simulink model "CubeX"  (R2016b)
settings: Solver=FixedStepAuto  StartTime=0.0  StopTime=10.0  RelTol=1e-3
values from neighbouring files (symbols this model uses):
  A = [0 0 0 0 0 0 0 0 0 0 283.190307038 0 ... (36 elements, 6x6)]    [K_lqr_3D.mat]
  C = [1 0 0 0 0 0 0 1 0 0 0 0 ... (36 elements, 6x6)]    [K_lqr_3D.mat]
  controller =     [K_lqr_3D.mat]
  deg_ = 0.0174532925199    [K_lqr_3D.mat]
  g = 9.81    [K_lqr_3D.mat]
  imu =     [K_lqr_3D.mat]
  K_lqr = [204.402503892 25.7626324054]    [K_lqr_3D.mat]
undefined symbols (not defined in the file or in its folder): CPHA_1Edge, CPOL_Low, Duplex, FirstBit_MSB, Full, Link, LQFP100, ST, STM32F407VG, STM32F4DISCOVERY
libraries: simulink x22, stm32f4_spi_lib x4, stm32f4_io_lib x2, stm32f4_adc_lib x1, cube_lib x1, stm32f4_device_config_lib x1, BC_USB x1
(part 2 of 3)

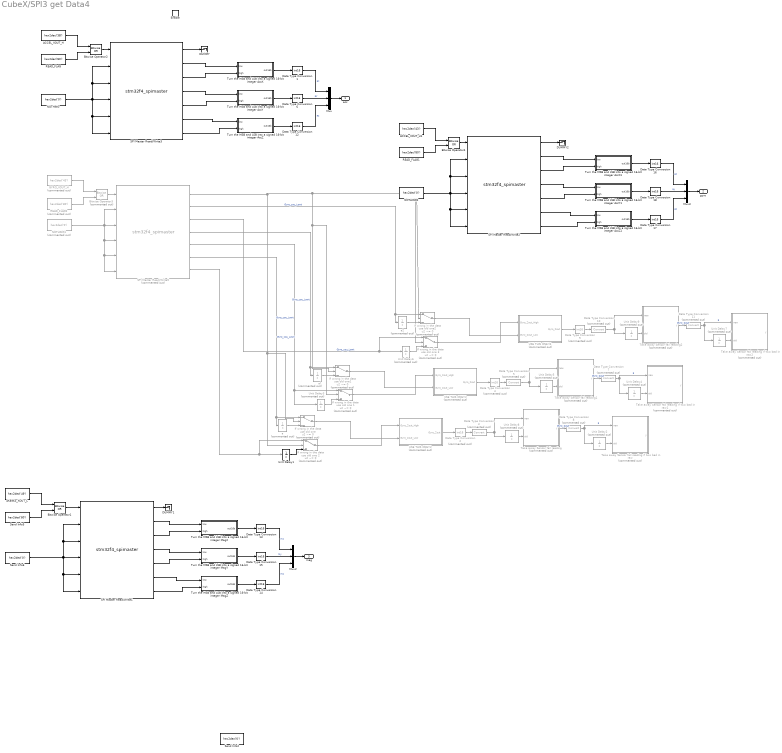
== system CubeX/SPI3 get Data4 ==
  Enable : EnablePort
  " a" : UnitDelay  Commented=on  SampleTime=-1
  " a1" : UnitDelay  Commented=on  SampleTime=-1
  " a2" : UnitDelay  Commented=on  SampleTime=-1
  ACCEL_XOUT_H : Constant  Value=hex2dec('3B')  OutDataTypeStr=uint8
  ACCEL_XOUT_H1 : Constant  Value=hex2dec('43')  OutDataTypeStr=uint8
  AK8963_XOUT_L : Constant  Value=hex2dec('49')  OutDataTypeStr=uint8
  Bitwise Operator1 : simulink/Logic and Bit Operations/Bitwise Operator  logicop=OR  UseBitMask=off  NumInputPorts=2  BitMask=bin2dec('11011001')  BitMaskRealWorld=Stored Integer
  Bitwise Operator2 : simulink/Logic and Bit Operations/Bitwise Operator  logicop=OR  UseBitMask=off  NumInputPorts=2  BitMask=bin2dec('11011001')  BitMaskRealWorld=Stored Integer
  Bitwise Operator3 : simulink/Logic and Bit Operations/Bitwise Operator  Commented=on  logicop=OR  UseBitMask=off  NumInputPorts=2  BitMask=bin2dec('11011001')  BitMaskRealWorld=Stored Integer
  Bitwise Operator4 : simulink/Logic and Bit Operations/Bitwise Operator  logicop=OR  UseBitMask=off  NumInputPorts=2  BitMask=bin2dec('11011001')  BitMaskRealWorld=Stored Integer
  DUMMY : Terminator
  DUMMY1 : Terminator
  DUMMY2 : Terminator
  Data Type Conversion{1,6,12..18} (9 alike) : DataTypeConversion  OutDataTypeStr=int16
  Data Type Conversion{3,5,7..8,10..11} (6 alike) : DataTypeConversion  Commented=on
  Data Type Conversion2 : DataTypeConversion  Commented=on  OutDataTypeStr=int16
  Data Type Conversion4 : DataTypeConversion  Commented=on  OutDataTypeStr=int16
  Data Type Conversion9 : DataTypeConversion  Commented=on  OutDataTypeStr=int16
  GYRO_XOUT_H : Constant  Commented=on  Value=hex2dec('43')  OutDataTypeStr=uint8
  If wrong in the data use old one : Switch  Commented=on  Criteria=u2 ~= 0
  If wrong in the data use old one 1 : Switch  Commented=on  Criteria=u2 ~= 0
  If wrong in the data use old one 2 : Switch  Commented=on  Criteria=u2 ~= 0
  If wrong in the data use old one 3 : Switch  Commented=on  Criteria=u2 ~= 0
  If wrong in the data use old one1 : Switch  Commented=on  Criteria=u2 ~= 0
  If wrong in the data use old one2 : Switch  Commented=on  Criteria=u2 ~= 0
  Mux : Mux  Inputs=3
  Mux2 : Mux  Inputs=3
  Mux3 : Mux  Inputs=3
  NOTHING : Constant  Value=hex2dec('0')  OutDataTypeStr=uint8
  NOTHING1 : Constant  Commented=on  Value=hex2dec('0')  OutDataTypeStr=uint8
  NOTHING2 : Constant  Value=hex2dec('0')  OutDataTypeStr=uint8
  READ_FLAG : Constant  Value=hex2dec('80')  OutDataTypeStr=uint8
  READ_FLAG1 : Constant  Value=hex2dec('80')  OutDataTypeStr=uint8
  READ_FLAG2 : Constant  Commented=on  Value=hex2dec('80')  OutDataTypeStr=uint8
  SPI Master Read/Write1 : S-Function  FunctionName=stm32f4_spimaster  Parameters=mode,configuration,module,datacount,inputtypearray,outputtypearray,confstr,sampletime,sampletimestr,blockid  SFunctionDeploymentMode=off  EnableBusSupport=off  mask(stm32f4_spimaster){configuration=Transaction, module=3, mode=Read/ Write, lastmodule=1, direction=Full-Duplex, dataformat=8bit/ FirstBit_MSB, prescaler=4, cpolcpha=CPOL_Low/ CPHA_1Edge, datacount=6, nssmode=Custom, nsspin=Not used, softnssport=E, softnsspin=0, sckpin=A5, misopin=A6, mosipin=A7, inputtypearray=[6 3 3 3 3 3 3], outputtypearray=[7 7 3 3 3 3 3 3], confstr=["SPI_Direction_2Lines_FullDuplex","8b","MSB","Low","1Edge","4","Soft","0","x","x","0","x","x","1","A","5","1","A","6","1","A","7","1","0","0","0","0","0","0","0","0","PP","0","UP"], sampletime=0.002, sampletimestr=0.002, blockid=SPI3getData4SPIMasterReadWrite1}
      mask prompts: module "SPI Module:"; lastmodule "Last module:"; dataformat "Data format:"; prescaler "Buad rate prescaler: Pclk/"; cpolcpha "Clock polarity (CPOL)/ Clock phase (CPHA):"; datacount "Data Read/Write count:"; nssmode "Slave/chip select (nSS, nCS) mode"; nsspin "Slave/chip select (nSS, nCS) pin"; softnssport "Slave/chip select port (nSS, nCS)"; softnsspin "Slave/chip select pin (nSS, nCS)"; sckpin "SCLK pin:"; misopin "MISO pin:"; mosipin "MOSI pin:"; inputtypearray "Input type array"; outputtypearray "Output type array"; confstr "Configuration string"; sampletime "Sample time (sec)"; sampletimestr "Compiled sample time (sec) in string"
      mask help:
      | Status:
      |  0 - Success.
      |  Otherwise - Fail.
      mask init:
      | stm32f4_spimaster_callback('init');
      mask Help: web(fullfile(waijungdocroot,'stm32f4_spimaster_readwrite.htm'), '-browser')
      mask TypeOptions configuration: Setup | Transaction
      mask Callback configuration: stm32f4_spimaster_callback('configuration');
      mask TypeOptions module: 1 | 2 | 3
      mask Callback module: stm32f4_spimaster_callback('module');
      mask TypeOptions mode: Read/ Write | Read | Write
      mask Callback mode: stm32f4_spimaster_callback('mode');
      mask TypeOptions direction: Full-Duplex | Half-Duplex_Tx | Half-Duplex_Rx
      mask Callback direction: stm32f4_spimaster_callback('direction');
      mask TypeOptions dataformat: 8bit/ FirstBit_MSB | 8bit/ FirstBit_LSB | 16bit/ FirstBit_MSB | 16bit/ FirstBit_LSB
      mask TypeOptions prescaler: 2 | 4 | 8 | 16 | 32 | 64 | 128 | 256
      mask TypeOptions cpolcpha: CPOL_Low/ CPHA_1Edge | CPOL_Low/ CPHA_2Edge | CPOL_High/ CPHA_1Edge | CPOL_High/ CPHA_2Edge
      mask Callback datacount: stm32f4_spimaster_callback('datacount');
      mask TypeOptions nssmode: Hardware | Software | Custom
      mask Callback nssmode: stm32f4_spimaster_callback('nssmode');
      mask TypeOptions nsspin: Not used | A4 | A15
      mask TypeOptions softnssport: A | B | C | D | E | F | G | H | I
      mask TypeOptions softnsspin: 0 | 1 | 2 | 3 | 4 | 5 | 6 | 7 | 8 | 9 | 10 | 11 | 12 | 13 | 14 | 15
      mask TypeOptions sckpin: Not used | A5 | B3
      mask TypeOptions misopin: Not used | A6 | B4
      mask TypeOptions mosipin: Not used | A7 | B5
      mask Callback confstr: stm32f4_spimaster_callback('confstr');
      mask Callback sampletime: stm32f4_spimaster_callback('sampletime');
      mask Callback sampletimestr: stm32f4_spimaster_callback('sampletimestr');
      mask Callback blockid: stm32f4_spimaster_callback('blockid');
      mask Display: text(0.5, 0.5, 'Module: SPI3 (Master)\nRead/ Write\nTs (sec): 0.002','ver','middle','hor','center');port_label('input', 1,'Wr0 (uint8)');port_label('input', 2,'Wr1 (uint8)');port_label('input', 3,'Wr2 (uint8)');port_label('input', 4,'Wr3 (uint8)');port_label('input', 5,'Wr4 (uint8)');port_label('input', 6,'Wr5 (uint8)');port_label('output', 1,'Status');port_label('output', 2,'Rd0 (uint8)');port_label('output', 3,'Rd1 (uint8)');port_label('output', 4,'Rd2 (uint8)');port_label('output', 5,'Rd3 (uint8)');port_label('output', 6,'Rd4 (uint8)');port_label('output', 7,'Rd5 (uint8)');
  SPI Master Read/Write2 : S-Function  FunctionName=stm32f4_spimaster  Parameters=mode,configuration,module,datacount,inputtypearray,outputtypearray,confstr,sampletime,sampletimestr,blockid  SFunctionDeploymentMode=off  EnableBusSupport=off  mask(stm32f4_spimaster){configuration=Transaction, module=3, mode=Read/ Write, lastmodule=1, direction=Full-Duplex, dataformat=8bit/ FirstBit_MSB, prescaler=4, cpolcpha=CPOL_Low/ CPHA_1Edge, datacount=6, nssmode=Custom, nsspin=Not used, softnssport=E, softnsspin=0, sckpin=A5, misopin=A6, mosipin=A7, inputtypearray=[6 3 3 3 3 3 3], outputtypearray=[7 7 3 3 3 3 3 3], confstr=["SPI_Direction_2Lines_FullDuplex","8b","MSB","Low","1Edge","4","Soft","0","x","x","0","x","x","1","A","5","1","A","6","1","A","7","1","0","0","0","0","0","0","0","0","PP","0","UP"], sampletime=-1, sampletimestr=Inf, blockid=SPI3getData4SPIMasterReadWrite2}
      mask prompts: module "SPI Module:"; lastmodule "Last module:"; dataformat "Data format:"; prescaler "Buad rate prescaler: Pclk/"; cpolcpha "Clock polarity (CPOL)/ Clock phase (CPHA):"; datacount "Data Read/Write count:"; nssmode "Slave/chip select (nSS, nCS) mode"; nsspin "Slave/chip select (nSS, nCS) pin"; softnssport "Slave/chip select port (nSS, nCS)"; softnsspin "Slave/chip select pin (nSS, nCS)"; sckpin "SCLK pin:"; misopin "MISO pin:"; mosipin "MOSI pin:"; inputtypearray "Input type array"; outputtypearray "Output type array"; confstr "Configuration string"; sampletime "Sample time (sec)"; sampletimestr "Compiled sample time (sec) in string"
      mask help:
      | Status:
      |  0 - Success.
      |  Otherwise - Fail.
      mask init:
      | stm32f4_spimaster_callback('init');
      mask Help: web(fullfile(waijungdocroot,'stm32f4_spimaster_readwrite.htm'), '-browser')
      mask TypeOptions configuration: Setup | Transaction
      mask Callback configuration: stm32f4_spimaster_callback('configuration');
      mask TypeOptions module: 1 | 2 | 3
      mask Callback module: stm32f4_spimaster_callback('module');
      mask TypeOptions mode: Read/ Write | Read | Write
      mask Callback mode: stm32f4_spimaster_callback('mode');
      mask TypeOptions direction: Full-Duplex | Half-Duplex_Tx | Half-Duplex_Rx
      mask Callback direction: stm32f4_spimaster_callback('direction');
      mask TypeOptions dataformat: 8bit/ FirstBit_MSB | 8bit/ FirstBit_LSB | 16bit/ FirstBit_MSB | 16bit/ FirstBit_LSB
      mask TypeOptions prescaler: 2 | 4 | 8 | 16 | 32 | 64 | 128 | 256
      mask TypeOptions cpolcpha: CPOL_Low/ CPHA_1Edge | CPOL_Low/ CPHA_2Edge | CPOL_High/ CPHA_1Edge | CPOL_High/ CPHA_2Edge
      mask Callback datacount: stm32f4_spimaster_callback('datacount');
      mask TypeOptions nssmode: Hardware | Software | Custom
      mask Callback nssmode: stm32f4_spimaster_callback('nssmode');
      mask TypeOptions nsspin: Not used | A4 | A15
      mask TypeOptions softnssport: A | B | C | D | E | F | G | H | I
      mask TypeOptions softnsspin: 0 | 1 | 2 | 3 | 4 | 5 | 6 | 7 | 8 | 9 | 10 | 11 | 12 | 13 | 14 | 15
      mask TypeOptions sckpin: Not used | A5 | B3
      mask TypeOptions misopin: Not used | A6 | B4
      mask TypeOptions mosipin: Not used | A7 | B5
      mask Callback confstr: stm32f4_spimaster_callback('confstr');
      mask Callback sampletime: stm32f4_spimaster_callback('sampletime');
      mask Callback sampletimestr: stm32f4_spimaster_callback('sampletimestr');
      mask Callback blockid: stm32f4_spimaster_callback('blockid');
      mask Display: text(0.5, 0.5, 'Module: SPI3 (Master)\nRead/ Write\nTs (sec): Inf','ver','middle','hor','center');port_label('input', 1,'Wr0 (uint8)');port_label('input', 2,'Wr1 (uint8)');port_label('input', 3,'Wr2 (uint8)');port_label('input', 4,'Wr3 (uint8)');port_label('input', 5,'Wr4 (uint8)');port_label('input', 6,'Wr5 (uint8)');port_label('output', 1,'Status');port_label('output', 2,'Rd0 (uint8)');port_label('output', 3,'Rd1 (uint8)');port_label('output', 4,'Rd2 (uint8)');port_label('output', 5,'Rd3 (uint8)');port_label('output', 6,'Rd4 (uint8)');port_label('output', 7,'Rd5 (uint8)');
  SPI Master Read/Write3 : S-Function  FunctionName=stm32f4_spimaster  Parameters=mode,configuration,module,datacount,inputtypearray,outputtypearray,confstr,sampletime,sampletimestr,blockid  SFunctionDeploymentMode=off  EnableBusSupport=off  mask(stm32f4_spimaster){configuration=Transaction, module=3, mode=Read/ Write, lastmodule=1, direction=Full-Duplex, dataformat=8bit/ FirstBit_MSB, prescaler=4, cpolcpha=CPOL_Low/ CPHA_1Edge, datacount=6, nssmode=Custom, nsspin=Not used, softnssport=E, softnsspin=0, sckpin=A5, misopin=A6, mosipin=A7, inputtypearray=[6 3 3 3 3 3 3], outputtypearray=[7 7 3 3 3 3 3 3], confstr=["SPI_Direction_2Lines_FullDuplex","8b","MSB","Low","1Edge","4","Soft","0","x","x","0","x","x","1","A","5","1","A","6","1","A","7","1","0","0","0","0","0","0","0","0","PP","0","UP"], sampletime=-1, sampletimestr=Inf, blockid=SPI3getData4SPIMasterReadWrite3}
      mask prompts: module "SPI Module:"; lastmodule "Last module:"; dataformat "Data format:"; prescaler "Buad rate prescaler: Pclk/"; cpolcpha "Clock polarity (CPOL)/ Clock phase (CPHA):"; datacount "Data Read/Write count:"; nssmode "Slave/chip select (nSS, nCS) mode"; nsspin "Slave/chip select (nSS, nCS) pin"; softnssport "Slave/chip select port (nSS, nCS)"; softnsspin "Slave/chip select pin (nSS, nCS)"; sckpin "SCLK pin:"; misopin "MISO pin:"; mosipin "MOSI pin:"; inputtypearray "Input type array"; outputtypearray "Output type array"; confstr "Configuration string"; sampletime "Sample time (sec)"; sampletimestr "Compiled sample time (sec) in string"
      mask help:
      | Status:
      |  0 - Success.
      |  Otherwise - Fail.
      mask init:
      | stm32f4_spimaster_callback('init');
      mask Help: web(fullfile(waijungdocroot,'stm32f4_spimaster_readwrite.htm'), '-browser')
      mask TypeOptions configuration: Setup | Transaction
      mask Callback configuration: stm32f4_spimaster_callback('configuration');
      mask TypeOptions module: 1 | 2 | 3
      mask Callback module: stm32f4_spimaster_callback('module');
      mask TypeOptions mode: Read/ Write | Read | Write
      mask Callback mode: stm32f4_spimaster_callback('mode');
      mask TypeOptions direction: Full-Duplex | Half-Duplex_Tx | Half-Duplex_Rx
      mask Callback direction: stm32f4_spimaster_callback('direction');
      mask TypeOptions dataformat: 8bit/ FirstBit_MSB | 8bit/ FirstBit_LSB | 16bit/ FirstBit_MSB | 16bit/ FirstBit_LSB
      mask TypeOptions prescaler: 2 | 4 | 8 | 16 | 32 | 64 | 128 | 256
      mask TypeOptions cpolcpha: CPOL_Low/ CPHA_1Edge | CPOL_Low/ CPHA_2Edge | CPOL_High/ CPHA_1Edge | CPOL_High/ CPHA_2Edge
      mask Callback datacount: stm32f4_spimaster_callback('datacount');
      mask TypeOptions nssmode: Hardware | Software | Custom
      mask Callback nssmode: stm32f4_spimaster_callback('nssmode');
      mask TypeOptions nsspin: Not used | A4 | A15
      mask TypeOptions softnssport: A | B | C | D | E | F | G | H | I
      mask TypeOptions softnsspin: 0 | 1 | 2 | 3 | 4 | 5 | 6 | 7 | 8 | 9 | 10 | 11 | 12 | 13 | 14 | 15
      mask TypeOptions sckpin: Not used | A5 | B3
      mask TypeOptions misopin: Not used | A6 | B4
      mask TypeOptions mosipin: Not used | A7 | B5
      mask Callback confstr: stm32f4_spimaster_callback('confstr');
      mask Callback sampletime: stm32f4_spimaster_callback('sampletime');
      mask Callback sampletimestr: stm32f4_spimaster_callback('sampletimestr');
      mask Callback blockid: stm32f4_spimaster_callback('blockid');
      mask Display: text(0.5, 0.5, 'Module: SPI3 (Master)\nRead/ Write\nTs (sec): Inf','ver','middle','hor','center');port_label('input', 1,'Wr0 (uint8)');port_label('input', 2,'Wr1 (uint8)');port_label('input', 3,'Wr2 (uint8)');port_label('input', 4,'Wr3 (uint8)');port_label('input', 5,'Wr4 (uint8)');port_label('input', 6,'Wr5 (uint8)');port_label('output', 1,'Status');port_label('output', 2,'Rd0 (uint8)');port_label('output', 3,'Rd1 (uint8)');port_label('output', 4,'Rd2 (uint8)');port_label('output', 5,'Rd3 (uint8)');port_label('output', 6,'Rd4 (uint8)');port_label('output', 7,'Rd5 (uint8)');
  SPI Master Read/Write5 : S-Function  Commented=on  FunctionName=stm32f4_spimaster  Parameters=mode,configuration,module,datacount,inputtypearray,outputtypearray,confstr,sampletime,sampletimestr,blockid  SFunctionDeploymentMode=off  EnableBusSupport=off  mask(stm32f4_spimaster){configuration=Transaction, module=3, mode=Read/ Write, lastmodule=1, direction=Full-Duplex, dataformat=8bit/ FirstBit_MSB, prescaler=4, cpolcpha=CPOL_Low/ CPHA_1Edge, datacount=6, nssmode=Custom, nsspin=Not used, softnssport=E, softnsspin=0, sckpin=A5, misopin=A6, mosipin=A7, inputtypearray=[6 3 3 3 3 3 3], outputtypearray=[7 7 3 3 3 3 3 3], confstr=["SPI_Direction_2Lines_FullDuplex","8b","MSB","Low","1Edge","4","Soft","0","x","x","0","x","x","1","A","5","1","A","6","1","A","7","1","0","0","0","0","0","0","0","0","PP","0","UP"], sampletime=-1, sampletimestr=Inf, blockid=SPI3getData4SPIMasterReadWrite5}
      mask prompts: module "SPI Module:"; lastmodule "Last module:"; dataformat "Data format:"; prescaler "Buad rate prescaler: Pclk/"; cpolcpha "Clock polarity (CPOL)/ Clock phase (CPHA):"; datacount "Data Read/Write count:"; nssmode "Slave/chip select (nSS, nCS) mode"; nsspin "Slave/chip select (nSS, nCS) pin"; softnssport "Slave/chip select port (nSS, nCS)"; softnsspin "Slave/chip select pin (nSS, nCS)"; sckpin "SCLK pin:"; misopin "MISO pin:"; mosipin "MOSI pin:"; inputtypearray "Input type array"; outputtypearray "Output type array"; confstr "Configuration string"; sampletime "Sample time (sec)"; sampletimestr "Compiled sample time (sec) in string"
      mask help:
      | Status:
      |  0 - Success.
      |  Otherwise - Fail.
      mask init:
      | stm32f4_spimaster_callback('init');
      mask Help: web(fullfile(waijungdocroot,'stm32f4_spimaster_readwrite.htm'), '-browser')
      mask TypeOptions configuration: Setup | Transaction
      mask Callback configuration: stm32f4_spimaster_callback('configuration');
      mask TypeOptions module: 1 | 2 | 3
      mask Callback module: stm32f4_spimaster_callback('module');
      mask TypeOptions mode: Read/ Write | Read | Write
      mask Callback mode: stm32f4_spimaster_callback('mode');
      mask TypeOptions direction: Full-Duplex | Half-Duplex_Tx | Half-Duplex_Rx
      mask Callback direction: stm32f4_spimaster_callback('direction');
      mask TypeOptions dataformat: 8bit/ FirstBit_MSB | 8bit/ FirstBit_LSB | 16bit/ FirstBit_MSB | 16bit/ FirstBit_LSB
      mask TypeOptions prescaler: 2 | 4 | 8 | 16 | 32 | 64 | 128 | 256
      mask TypeOptions cpolcpha: CPOL_Low/ CPHA_1Edge | CPOL_Low/ CPHA_2Edge | CPOL_High/ CPHA_1Edge | CPOL_High/ CPHA_2Edge
      mask Callback datacount: stm32f4_spimaster_callback('datacount');
      mask TypeOptions nssmode: Hardware | Software | Custom
      mask Callback nssmode: stm32f4_spimaster_callback('nssmode');
      mask TypeOptions nsspin: Not used | A4 | A15
      mask TypeOptions softnssport: A | B | C | D | E | F | G | H | I
      mask TypeOptions softnsspin: 0 | 1 | 2 | 3 | 4 | 5 | 6 | 7 | 8 | 9 | 10 | 11 | 12 | 13 | 14 | 15
      mask TypeOptions sckpin: Not used | A5 | B3
      mask TypeOptions misopin: Not used | A6 | B4
      mask TypeOptions mosipin: Not used | A7 | B5
      mask Callback confstr: stm32f4_spimaster_callback('confstr');
      mask Callback sampletime: stm32f4_spimaster_callback('sampletime');
      mask Callback sampletimestr: stm32f4_spimaster_callback('sampletimestr');
      mask Callback blockid: stm32f4_spimaster_callback('blockid');
      mask Display: text(0.5, 0.5, 'Module: SPI3 (Master)\nRead/ Write\nTs (sec): Inf','ver','middle','hor','center');port_label('input', 1,'Wr0 (uint8)');port_label('input', 2,'Wr1 (uint8)');port_label('input', 3,'Wr2 (uint8)');port_label('input', 4,'Wr3 (uint8)');port_label('input', 5,'Wr4 (uint8)');port_label('input', 6,'Wr5 (uint8)');port_label('output', 1,'Status');port_label('output', 2,'Rd0 (uint8)');port_label('output', 3,'Rd1 (uint8)');port_label('output', 4,'Rd2 (uint8)');port_label('output', 5,'Rd3 (uint8)');port_label('output', 6,'Rd4 (uint8)');port_label('output', 7,'Rd5 (uint8)');
  Send Info2 : Constant  Value=hex2dec('0')  OutDataTypeStr=uint8
  Send Info5 : Constant  Value=hex2dec('80')  OutDataTypeStr=uint8
  Send Info6 : Constant  Value=hex2dec('0')  OutDataTypeStr=uint8
  Take away Sensor fail reading : MATLAB Function  Commented=on  TreatAsAtomicUnit=on
  Take away Sensor fail reading if two bad in raw : MATLAB Function  Commented=on  TreatAsAtomicUnit=on
  Take away Sensor fail reading if two bad in raw1 : MATLAB Function  Commented=on  TreatAsAtomicUnit=on
  Take away Sensor fail reading if two bad in raw2 : MATLAB Function  Commented=on  TreatAsAtomicUnit=on
  Take away Sensor fail reading1 : MATLAB Function  Commented=on  TreatAsAtomicUnit=on
  Take away Sensor fail reading2 : MATLAB Function  Commented=on  TreatAsAtomicUnit=on
  Turn the MSB and LSB into a signed 16-bit integer AccX : Subsystem
  Turn the MSB and LSB into a signed 16-bit integer AccX1 : Subsystem
  Turn the MSB and LSB into a signed 16-bit integer AccY : Subsystem
  Turn the MSB and LSB into a signed 16-bit integer AccY1 : Subsystem
  Turn the MSB and LSB into a signed 16-bit integer AccZ : Subsystem
  Turn the MSB and LSB into a signed 16-bit integer AccZ1 : Subsystem
  Turn the MSB and LSB into a signed 16-bit integer MagX : Subsystem
  Turn the MSB and LSB into a signed 16-bit integer MagY : Subsystem
  Turn the MSB and LSB into a signed 16-bit integer MagZ : Subsystem
  USE THIS ONE!!2 : Subsystem  Commented=on
  USE THIS ONE!!3 : Subsystem  Commented=on
  USE THIS ONE!!4 : Subsystem  Commented=on
  Unit Delay1 : UnitDelay  SampleTime=-1
  Unit Delay{2,4..5,7..9} (6 alike) : UnitDelay  Commented=on  InitialCondition=-40.45  SampleTime=-1
  Unit Delay3 : UnitDelay  Commented=on  SampleTime=-1
  Unit Delay6 : UnitDelay  Commented=on  SampleTime=-1
  acc : Outport
  gyro : Outport  Port=2
  mag : Outport  Port=3
  wires:
  Bitwise Operator3/1 -> SPI Master Read/Write5/1
  ACCEL_XOUT_H/1 -> Bitwise Operator2/1
  GYRO_XOUT_H/1 -> Bitwise Operator3/1
  READ_FLAG2/1 -> Bitwise Operator3/2
  Bitwise Operator2/1 -> SPI Master Read/Write3/1
  READ_FLAG/1 -> Bitwise Operator2/2
  NOTHING1/1 -> SPI Master Read/Write5/2, SPI Master Read/Write5/6, SPI Master Read/Write5/5, SPI Master Read/Write5/4, SPI Master Read/Write5/3
  SPI Master Read/Write3/1 -> DUMMY/1
  USE THIS ONE!!2/1(Gyro_Zout) -> Data Type Conversion2/1
  Data Type Conversion2/1 -> Data Type Conversion3/1
  SPI Master Read/Write5/6 -> " a"/1, If wrong in the data use old one/1  "Gyro_zou_Lowt"
  " a"/1 -> If wrong in the data use old one/3
  SPI Master Read/Write5/7 -> If wrong in the data use old one 2/1, Unit Delay1/1
  Unit Delay1/1 -> If wrong in the data use old one 2/3
  If wrong in the data use old one/1 -> USE THIS ONE!!2/2(Gyro_Zout_Low)
  If wrong in the data use old one 2/1 -> USE THIS ONE!!2/1("Gyro_Zout_High ")
  Unit Delay8/1 -> Take away Sensor fail reading/2(old)
  Take away Sensor fail reading/1(y) -> Data Type Conversion8/1  "Gyro_Zout"
  Unit Delay2/1 -> Take away Sensor fail reading if two bad in raw/2(old)
  Data Type Conversion8/1 -> Unit Delay2/1, Take away Sensor fail reading if two bad in raw/1(new)  "3"
  Data Type Conversion3/1 -> Take away Sensor fail reading/1(new), Unit Delay8/1
  SPI Master Read/Write5/3 -> If wrong in the data use old one 3/1, Unit Delay6/1  "Gyro_zou_Lowt"
  SPI Master Read/Write5/5 -> Unit Delay3/1, If wrong in the data use old one 1/1  "Gyro_zou_Lowt"
  USE THIS ONE!!3/1(Gyro_Zout) -> Data Type Conversion4/1
  Data Type Conversion4/1 -> Data Type Conversion5/1
  SPI Master Read/Write5/4 -> " a1"/1, If wrong in the data use old one1/1  "Gyro_zou_Lowt"
  " a1"/1 -> If wrong in the data use old one1/3
  Unit Delay3/1 -> If wrong in the data use old one 1/3
  If wrong in the data use old one1/1 -> USE THIS ONE!!3/2(Gyro_Zout_Low)
  If wrong in the data use old one 1/1 -> USE THIS ONE!!3/1("Gyro_Zout_High ")
  Unit Delay5/1 -> Take away Sensor fail reading1/2(old)
  Take away Sensor fail reading1/1(y) -> Data Type Conversion7/1  "Gyro_Zout"
  Unit Delay4/1 -> Take away Sensor fail reading if two bad in raw1/2(old)
  Data Type Conversion7/1 -> Unit Delay4/1, Take away Sensor fail reading if two bad in raw1/1(new)  "3"
  Data Type Conversion5/1 -> Take away Sensor fail reading1/1(new), Unit Delay5/1
  USE THIS ONE!!4/1(Gyro_Zout) -> Data Type Conversion9/1
  Data Type Conversion9/1 -> Data Type Conversion10/1
  SPI Master Read/Write5/2 -> " a2"/1, If wrong in the data use old one2/1  "Gyro_zou_Lowt"
  " a2"/1 -> If wrong in the data use old one2/3
  Unit Delay6/1 -> If wrong in the data use old one 3/3
  If wrong in the data use old one2/1 -> USE THIS ONE!!4/2(Gyro_Zout_Low)
  If wrong in the data use old one 3/1 -> USE THIS ONE!!4/1("Gyro_Zout_High ")
  Unit Delay9/1 -> Take away Sensor fail reading2/2(old)
  Take away Sensor fail reading2/1(y) -> Data Type Conversion11/1  "Gyro_Zout"
  Unit Delay7/1 -> Take away Sensor fail reading if two bad in raw2/2(old)
  Data Type Conversion11/1 -> Unit Delay7/1, Take away Sensor fail reading if two bad in raw2/1(new)  "3"
  Data Type Conversion10/1 -> Take away Sensor fail reading2/1(new), Unit Delay9/1
  SPI Master Read/Write5/1 -> If wrong in the data use old one2/2, If wrong in the data use old one 3/2, If wrong in the data use old one 1/2, If wrong in the data use old one1/2, If wrong in the data use old one 2/2, If wrong in the data use old one/2
  NOTHING/1 -> SPI Master Read/Write3/2, SPI Master Read/Write3/3, SPI Master Read/Write3/4, SPI Master Read/Write3/5, SPI Master Read/Write3/6
  Mux/1 -> acc/1
  Turn the MSB and LSB into a signed 16-bit integer AccX/1(out16b) -> Data Type Conversion1/1
  Turn the MSB and LSB into a signed 16-bit integer AccY/1(out16b) -> Data Type Conversion6/1
  SPI Master Read/Write3/6 -> Turn the MSB and LSB into a signed 16-bit integer AccZ/1(low)
  SPI Master Read/Write3/7 -> Turn the MSB and LSB into a signed 16-bit integer AccZ/2(high)
  SPI Master Read/Write3/2 -> Turn the MSB and LSB into a signed 16-bit integer AccX/1(low)
  SPI Master Read/Write3/3 -> Turn the MSB and LSB into a signed 16-bit integer AccX/2(high)
  SPI Master Read/Write3/4 -> Turn the MSB and LSB into a signed 16-bit integer AccY/1(low)
  SPI Master Read/Write3/5 -> Turn the MSB and LSB into a signed 16-bit integer AccY/2(high)
  Turn the MSB and LSB into a signed 16-bit integer AccZ/1(out16b) -> Data Type Conversion12/1
  Data Type Conversion1/1 -> Mux/1  "ax"
  Data Type Conversion6/1 -> Mux/2  "ay"
  Data Type Conversion12/1 -> Mux/3  "az"
  AK8963_XOUT_L/1 -> Bitwise Operator1/1
  Bitwise Operator1/1 -> SPI Master Read/Write1/1
  Send Info5/1 -> Bitwise Operator1/2
  SPI Master Read/Write1/1 -> DUMMY1/1
  Send Info6/1 -> SPI Master Read/Write1/2, SPI Master Read/Write1/3, SPI Master Read/Write1/4, SPI Master Read/Write1/5, SPI Master Read/Write1/6
  Mux2/1 -> mag/1
  Turn the MSB and LSB into a signed 16-bit integer MagX/1(out16b) -> Data Type Conversion13/1
  Turn the MSB and LSB into a signed 16-bit integer MagY/1(out16b) -> Data Type Conversion15/1
  SPI Master Read/Write1/6 -> Turn the MSB and LSB into a signed 16-bit integer MagZ/1(low)
  SPI Master Read/Write1/7 -> Turn the MSB and LSB into a signed 16-bit integer MagZ/2(high)
  SPI Master Read/Write1/2 -> Turn the MSB and LSB into a signed 16-bit integer MagX/1(low)
  SPI Master Read/Write1/3 -> Turn the MSB and LSB into a signed 16-bit integer MagX/2(high)
  SPI Master Read/Write1/4 -> Turn the MSB and LSB into a signed 16-bit integer MagY/1(low)
  SPI Master Read/Write1/5 -> Turn the MSB and LSB into a signed 16-bit integer MagY/2(high)
  Turn the MSB and LSB into a signed 16-bit integer MagZ/1(out16b) -> Data Type Conversion14/1
  Data Type Conversion13/1 -> Mux2/1  "mx"
  Data Type Conversion15/1 -> Mux2/2  "my"
  Data Type Conversion14/1 -> Mux2/3  "mz"
  ACCEL_XOUT_H1/1 -> Bitwise Operator4/1
  Bitwise Operator4/1 -> SPI Master Read/Write2/1
  READ_FLAG1/1 -> Bitwise Operator4/2
  SPI Master Read/Write2/1 -> DUMMY2/1
  NOTHING2/1 -> SPI Master Read/Write2/2, SPI Master Read/Write2/3, SPI Master Read/Write2/4, SPI Master Read/Write2/5, SPI Master Read/Write2/6
  Mux3/1 -> gyro/1
  Turn the MSB and LSB into a signed 16-bit integer AccX1/1(out16b) -> Data Type Conversion16/1
  Turn the MSB and LSB into a signed 16-bit integer AccY1/1(out16b) -> Data Type Conversion18/1
  SPI Master Read/Write2/6 -> Turn the MSB and LSB into a signed 16-bit integer AccZ1/1(low)
  SPI Master Read/Write2/7 -> Turn the MSB and LSB into a signed 16-bit integer AccZ1/2(high)
  SPI Master Read/Write2/2 -> Turn the MSB and LSB into a signed 16-bit integer AccX1/1(low)
  SPI Master Read/Write2/3 -> Turn the MSB and LSB into a signed 16-bit integer AccX1/2(high)
  SPI Master Read/Write2/4 -> Turn the MSB and LSB into a signed 16-bit integer AccY1/1(low)
  SPI Master Read/Write2/5 -> Turn the MSB and LSB into a signed 16-bit integer AccY1/2(high)
  Turn the MSB and LSB into a signed 16-bit integer AccZ1/1(out16b) -> Data Type Conversion17/1
  Data Type Conversion16/1 -> Mux3/1  "ax"
  Data Type Conversion18/1 -> Mux3/2  "ay"
  Data Type Conversion17/1 -> Mux3/3  "az"

== system CubeX/State feedback controller(LQR) ==
  note: State feedback
      |
      | u = -Kx
  x : Inport
  Bus Selector2 : BusSelector  OutputSignals=cube_angle,cube_angular_velocity,motorStates.current
  Gain : Gain  Gain=-K_lqr  Multiplication=Matrix(K*u) (u vector)
  Mux : Mux  Inputs=3
  u : Outport
  wires:
  x/1 -> Bus Selector2/1
  Mux/1 -> Gain/1
  Gain/1 -> u/1  "[k_T*i]"
  Bus Selector2/1 -> Mux/1  "<cube_angle>"
  Bus Selector2/2 -> Mux/2  "<cube_angular_velocity>"
  Bus Selector2/3 -> Mux/3  "<current>"

== system CubeX/Subsystem ==
  acc_raw : Inport
  gyro_raw : Inport  Port=2
  Raw sensor value to SI units Accelometer : Gain  Gain=1 / imu.a_scaling * g
  Raw sensor value to SI units Gyroscope : Gain  Gain=1 / imu.w_scaling * deg_
  acc : Outport
  gyro : Outport  Port=2
  wires:
  gyro_raw/1 -> Raw sensor value to SI units Gyroscope/1
  Raw sensor value to SI units Accelometer/1 -> acc/1
  Raw sensor value to SI units Gyroscope/1 -> gyro/1
  acc_raw/1 -> Raw sensor value to SI units Accelometer/1

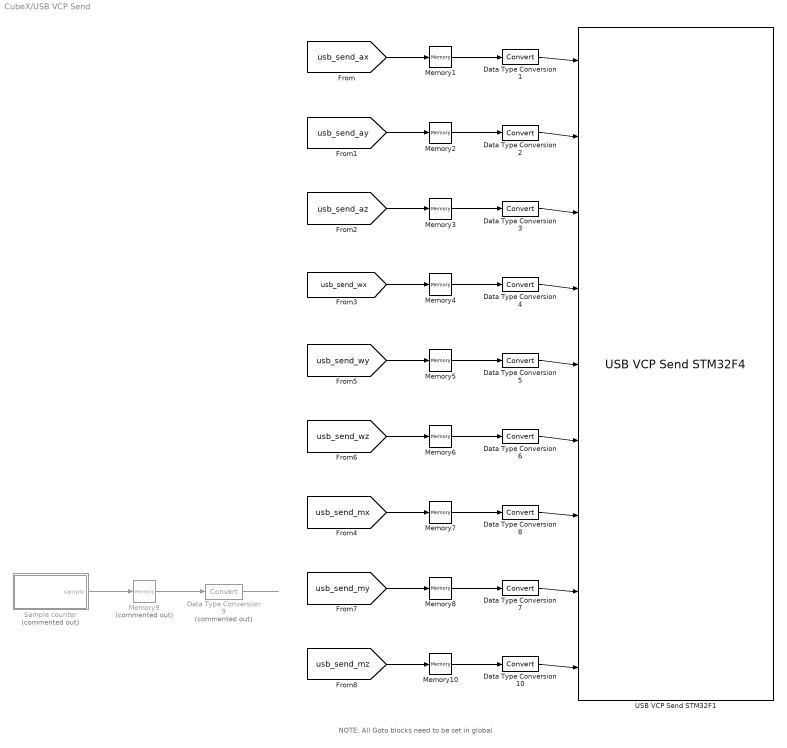
== system CubeX/USB VCP Send ==
  note: NOTE: All Goto blocks need to be set in global
  Data Type Conversion{1..8,10} (9 alike) : DataTypeConversion
  Data Type Conversion9 : DataTypeConversion  Commented=on
  Memory{1..8,10} (9 alike) : Memory  InheritSampleTime=on
  Memory9 : Memory  Commented=on  InheritSampleTime=on
  Sample counter : MATLAB Function  Commented=on  TreatAsAtomicUnit=on
  USB VCP Send STM32F1 : BC_USB/USB VCP Send STM32F4  speed="USB 1.1   12Mbit/s"  data_size=2048 Bytes  header_data='0E 0E'  binary_data='double double double double double double double double double'  terminator_data='0A 0A'  sampletime=0.002
  wires:
  Memory7/1 -> Data Type Conversion8/1
  Data Type Conversion8/1 -> USB VCP Send STM32F1/7
  Data Type Conversion1/1 -> USB VCP Send STM32F1/1
  Memory2/1 -> Data Type Conversion2/1
  Memory1/1 -> Data Type Conversion1/1
  [usb_send_ax] -> Memory1/1
  Data Type Conversion2/1 -> USB VCP Send STM32F1/2
  Memory6/1 -> Data Type Conversion6/1
  Data Type Conversion3/1 -> USB VCP Send STM32F1/3
  [usb_send_ay] -> Memory2/1
  [usb_send_az] -> Memory3/1
  Memory3/1 -> Data Type Conversion3/1
  Memory4/1 -> Data Type Conversion4/1
  [usb_send_wx] -> Memory4/1
  Data Type Conversion4/1 -> USB VCP Send STM32F1/4
  Memory5/1 -> Data Type Conversion5/1
  Data Type Conversion5/1 -> USB VCP Send STM32F1/5
  Data Type Conversion6/1 -> USB VCP Send STM32F1/6
  [usb_send_wy] -> Memory5/1
  [usb_send_mx] -> Memory7/1
  [usb_send_wz] -> Memory6/1
  Memory9/1 -> Data Type Conversion9/1
  Sample counter/1(sample) -> Memory9/1
  Data Type Conversion9/1 -> ?
  Memory8/1 -> Data Type Conversion7/1
  Data Type Conversion7/1 -> USB VCP Send STM32F1/8
  [usb_send_my] -> Memory8/1
  Memory10/1 -> Data Type Conversion10/1
  Data Type Conversion10/1 -> USB VCP Send STM32F1/9
  [usb_send_mz] -> Memory10/1

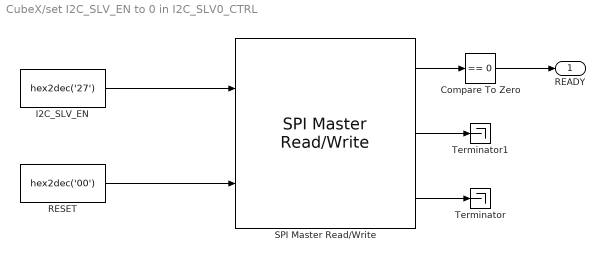
== system CubeX/set I2C_SLV_EN to 0 in I2C_SLV0_CTRL ==
  Compare To Zero : simulink/Logic and Bit Operations/Compare To Zero  relop===  OutDataTypeStr=boolean
  "I2C_SLV_EN " : Constant  Value=hex2dec('27')  OutDataTypeStr=uint8
  RESET : Constant  Value=hex2dec('00')  OutDataTypeStr=uint8
  SPI Master Read/Write : stm32f4_spi_lib/SPI Master Read//Write  configuration=Transaction  module=3  mode=Read/ Write  lastmodule=1  direction=Full-Duplex  dataformat=8bit/ FirstBit_MSB  prescaler=4  cpolcpha=CPOL_Low/ CPHA_1Edge  datacount=2  nssmode=Custom  nsspin=Not used  softnssport=E  softnsspin=0  sckpin=A5  misopin=A6  mosipin=A7  inputtypearray=[2 3 3]  outputtypearray=[3 7 3 3]  confstr="[\"SPI_Direction_2Lines_FullDuplex\",\"8b\",\"MSB\",\"Low\",\"1Edge\",\"4\",\"Soft\",\"0\",\"x\",\"x\",\"0\",\"x\",\"x\",\"1\",\"A\",\"5\",\"1\",\"A\",\"6\",\"1\",\"A\",\"7\",\"1\",\"0\",\"0\",\"0\",\"0\",\"0\",\"0\",\"0\",\"0\",\"PP\",\"0\",\"UP\"]"  sampletime=0.002  sampletimestr=0.002  blockid=setI2C_SLV_ENto0inI2C_SLV0_CTRLSPIMasterReadWrite
  Terminator : Terminator
  Terminator1 : Terminator
  READY : Outport
  wires:
  "I2C_SLV_EN "/1 -> SPI Master Read/Write/1
  RESET/1 -> SPI Master Read/Write/2
  SPI Master Read/Write/3 -> Terminator/1
  SPI Master Read/Write/1 -> Compare To Zero/1
  SPI Master Read/Write/2 -> Terminator1/1
  Compare To Zero/1 -> READY/1

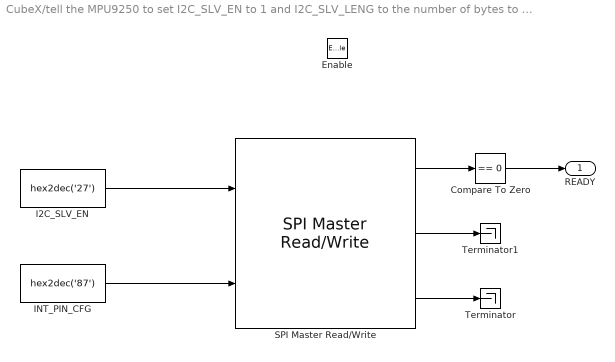
== system CubeX/tell the MPU9250 to set I2C_SLV_EN to 1 and I2C_SLV_LENG to the number of bytes to be transferred (1) in I2C_SLV0_CTRL ==
  Enable : EnablePort  StatesWhenEnabling=reset
  Compare To Zero : simulink/Logic and Bit Operations/Compare To Zero  relop===  OutDataTypeStr=boolean
  "I2C_SLV_EN " : Constant  Value=hex2dec('27')  OutDataTypeStr=uint8
  INT_PIN_CFG : Constant  Value=hex2dec('87')  OutDataTypeStr=uint8
  SPI Master Read/Write : stm32f4_spi_lib/SPI Master Read//Write  configuration=Transaction  module=3  mode=Read/ Write  lastmodule=1  direction=Full-Duplex  dataformat=8bit/ FirstBit_MSB  prescaler=4  cpolcpha=CPOL_Low/ CPHA_1Edge  datacount=2  nssmode=Custom  nsspin=Not used  softnssport=E  softnsspin=0  sckpin=A5  misopin=A6  mosipin=A7  inputtypearray=[2 3 3]  outputtypearray=[3 7 3 3]  confstr="[\"SPI_Direction_2Lines_FullDuplex\",\"8b\",\"MSB\",\"Low\",\"1Edge\",\"4\",\"Soft\",\"0\",\"x\",\"x\",\"0\",\"x\",\"x\",\"1\",\"A\",\"5\",\"1\",\"A\",\"6\",\"1\",\"A\",\"7\",\"1\",\"0\",\"0\",\"0\",\"0\",\"0\",\"0\",\"0\",\"0\",\"PP\",\"0\",\"UP\"]"  sampletime=0.002  sampletimestr=0.002  blockid=telltheMPU9250tosetI2C_SLV_ENto1andI2C_SLV_LENGtothenumberofbytestobetransferred1inI2C_SLV0_CTRLSPIMasterReadWrite
  Terminator : Terminator
  Terminator1 : Terminator
  READY : Outport
  wires:
  SPI Master Read/Write/1 -> Compare To Zero/1
  Compare To Zero/1 -> READY/1
  SPI Master Read/Write/3 -> Terminator/1
  SPI Master Read/Write/2 -> Terminator1/1
  "I2C_SLV_EN "/1 -> SPI Master Read/Write/1
  INT_PIN_CFG/1 -> SPI Master Read/Write/2

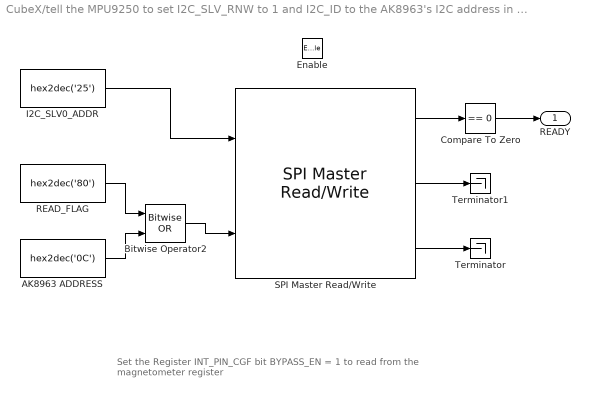
== system CubeX/tell the MPU9250 to set I2C_SLV_RNW to 1 and I2C_ID to the AK8963's I2C address in I2C_SLV0_ADDR ==
  note: Set the Register INT_PIN_CGF bit BYPASS_EN = 1 to read from
      | the magnetometer register
  Enable : EnablePort  StatesWhenEnabling=reset
  AK8963 ADDRESS : Constant  Value=hex2dec('0C')  OutDataTypeStr=uint8
  Bitwise Operator2 : simulink/Logic and Bit Operations/Bitwise Operator  logicop=OR  UseBitMask=off  NumInputPorts=2  BitMask=bin2dec('11011001')  BitMaskRealWorld=Stored Integer
  Compare To Zero : simulink/Logic and Bit Operations/Compare To Zero  relop===  OutDataTypeStr=boolean
  I2C_SLV0_ADDR : Constant  Value=hex2dec('25')  OutDataTypeStr=uint8
  READ_FLAG : Constant  Value=hex2dec('80')  OutDataTypeStr=uint8
  SPI Master Read/Write : stm32f4_spi_lib/SPI Master Read//Write  configuration=Transaction  module=3  mode=Read/ Write  lastmodule=1  direction=Full-Duplex  dataformat=8bit/ FirstBit_MSB  prescaler=4  cpolcpha=CPOL_Low/ CPHA_1Edge  datacount=2  nssmode=Custom  nsspin=Not used  softnssport=E  softnsspin=0  sckpin=A5  misopin=A6  mosipin=A7  inputtypearray=[2 3 3]  outputtypearray=[3 7 3 3]  confstr="[\"SPI_Direction_2Lines_FullDuplex\",\"8b\",\"MSB\",\"Low\",\"1Edge\",\"4\",\"Soft\",\"0\",\"x\",\"x\",\"0\",\"x\",\"x\",\"1\",\"A\",\"5\",\"1\",\"A\",\"6\",\"1\",\"A\",\"7\",\"1\",\"0\",\"0\",\"0\",\"0\",\"0\",\"0\",\"0\",\"0\",\"PP\",\"0\",\"UP\"]"  sampletime=0.002  sampletimestr=0.002  blockid=telltheMPU9250tosetI2C_SLV_RNWto1andI2C_IDtotheAK8963sI2CaddressinI2C_SLV0_ADDRSPIMasterReadWrite
  Terminator : Terminator
  Terminator1 : Terminator
  READY : Outport
  wires:
  I2C_SLV0_ADDR/1 -> SPI Master Read/Write/1
  READ_FLAG/1 -> Bitwise Operator2/1
  SPI Master Read/Write/1 -> Compare To Zero/1
  Compare To Zero/1 -> READY/1
  SPI Master Read/Write/2 -> Terminator1/1
  SPI Master Read/Write/3 -> Terminator/1
  Bitwise Operator2/1 -> SPI Master Read/Write/2
  AK8963 ADDRESS/1 -> Bitwise Operator2/2

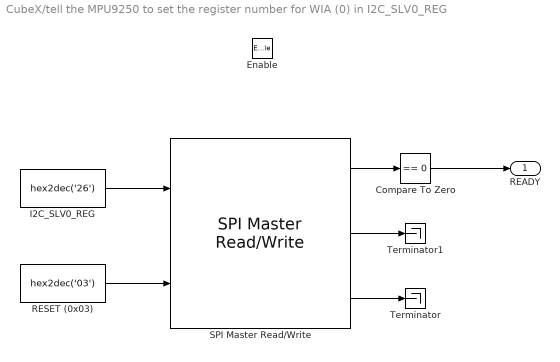
== system CubeX/tell the MPU9250 to set the register number for WIA (0) in I2C_SLV0_REG ==
  Enable : EnablePort  StatesWhenEnabling=reset
  Compare To Zero : simulink/Logic and Bit Operations/Compare To Zero  relop===  OutDataTypeStr=boolean
  I2C_SLV0_REG : Constant  Value=hex2dec('26')  OutDataTypeStr=uint8
  RESET (0x03) : Constant  Value=hex2dec('03')  OutDataTypeStr=uint8
  SPI Master Read/Write : stm32f4_spi_lib/SPI Master Read//Write  configuration=Transaction  module=3  mode=Read/ Write  lastmodule=1  direction=Full-Duplex  dataformat=8bit/ FirstBit_MSB  prescaler=4  cpolcpha=CPOL_Low/ CPHA_1Edge  datacount=2  nssmode=Custom  nsspin=Not used  softnssport=E  softnsspin=0  sckpin=A5  misopin=A6  mosipin=A7  inputtypearray=[2 3 3]  outputtypearray=[3 7 3 3]  confstr="[\"SPI_Direction_2Lines_FullDuplex\",\"8b\",\"MSB\",\"Low\",\"1Edge\",\"4\",\"Soft\",\"0\",\"x\",\"x\",\"0\",\"x\",\"x\",\"1\",\"A\",\"5\",\"1\",\"A\",\"6\",\"1\",\"A\",\"7\",\"1\",\"0\",\"0\",\"0\",\"0\",\"0\",\"0\",\"0\",\"0\",\"PP\",\"0\",\"UP\"]"  sampletime=0.002  sampletimestr=0.002  blockid=telltheMPU9250tosettheregisternumberforWIA0inI2C_SLV0_REGSPIMasterReadWrite
  Terminator : Terminator
  Terminator1 : Terminator
  READY : Outport
  wires:
  SPI Master Read/Write/1 -> Compare To Zero/1
  I2C_SLV0_REG/1 -> SPI Master Read/Write/1
  Compare To Zero/1 -> READY/1
  SPI Master Read/Write/3 -> Terminator/1
  RESET (0x03)/1 -> SPI Master Read/Write/2
  SPI Master Read/Write/2 -> Terminator1/1

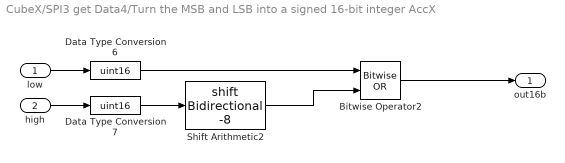
== system CubeX/SPI3 get Data4/Turn the MSB and LSB into a signed 16-bit integer AccX ==
  low : Inport
  high : Inport  Port=2
  Bitwise Operator2 : simulink/Logic and Bit Operations/Bitwise Operator  logicop=OR  UseBitMask=off  NumInputPorts=2  BitMask=bin2dec('11011001')  BitMaskRealWorld=Stored Integer
  Data Type Conversion6 : DataTypeConversion  OutDataTypeStr=uint16
  Data Type Conversion7 : DataTypeConversion  OutDataTypeStr=uint16
  Shift Arithmetic2 : ArithShift  BitShiftNumber=-8
  out16b : Outport
  wires:
  low/1 -> Data Type Conversion6/1
  Bitwise Operator2/1 -> out16b/1
  high/1 -> Data Type Conversion7/1
  Data Type Conversion7/1 -> Shift Arithmetic2/1
  Shift Arithmetic2/1 -> Bitwise Operator2/2
  Data Type Conversion6/1 -> Bitwise Operator2/1

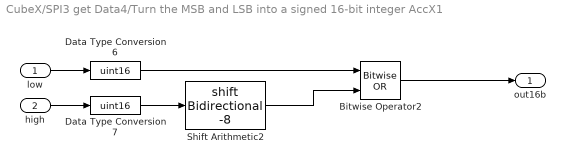
== system CubeX/SPI3 get Data4/Turn the MSB and LSB into a signed 16-bit integer AccX1 ==
  low : Inport
  high : Inport  Port=2
  Bitwise Operator2 : simulink/Logic and Bit Operations/Bitwise Operator  logicop=OR  UseBitMask=off  NumInputPorts=2  BitMask=bin2dec('11011001')  BitMaskRealWorld=Stored Integer
  Data Type Conversion6 : DataTypeConversion  OutDataTypeStr=uint16
  Data Type Conversion7 : DataTypeConversion  OutDataTypeStr=uint16
  Shift Arithmetic2 : ArithShift  BitShiftNumber=-8
  out16b : Outport
  wires:
  low/1 -> Data Type Conversion6/1
  Bitwise Operator2/1 -> out16b/1
  high/1 -> Data Type Conversion7/1
  Data Type Conversion7/1 -> Shift Arithmetic2/1
  Shift Arithmetic2/1 -> Bitwise Operator2/2
  Data Type Conversion6/1 -> Bitwise Operator2/1

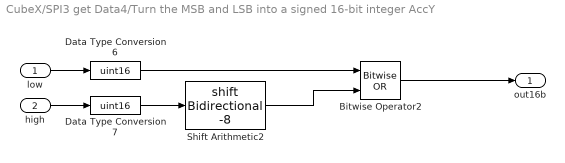
== system CubeX/SPI3 get Data4/Turn the MSB and LSB into a signed 16-bit integer AccY ==
  low : Inport
  high : Inport  Port=2
  Bitwise Operator2 : simulink/Logic and Bit Operations/Bitwise Operator  logicop=OR  UseBitMask=off  NumInputPorts=2  BitMask=bin2dec('11011001')  BitMaskRealWorld=Stored Integer
  Data Type Conversion6 : DataTypeConversion  OutDataTypeStr=uint16
  Data Type Conversion7 : DataTypeConversion  OutDataTypeStr=uint16
  Shift Arithmetic2 : ArithShift  BitShiftNumber=-8
  out16b : Outport
  wires:
  low/1 -> Data Type Conversion6/1
  Bitwise Operator2/1 -> out16b/1
  high/1 -> Data Type Conversion7/1
  Data Type Conversion7/1 -> Shift Arithmetic2/1
  Shift Arithmetic2/1 -> Bitwise Operator2/2
  Data Type Conversion6/1 -> Bitwise Operator2/1

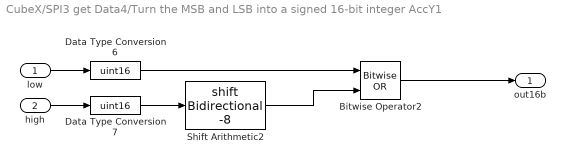
== system CubeX/SPI3 get Data4/Turn the MSB and LSB into a signed 16-bit integer AccY1 ==
  low : Inport
  high : Inport  Port=2
  Bitwise Operator2 : simulink/Logic and Bit Operations/Bitwise Operator  logicop=OR  UseBitMask=off  NumInputPorts=2  BitMask=bin2dec('11011001')  BitMaskRealWorld=Stored Integer
  Data Type Conversion6 : DataTypeConversion  OutDataTypeStr=uint16
  Data Type Conversion7 : DataTypeConversion  OutDataTypeStr=uint16
  Shift Arithmetic2 : ArithShift  BitShiftNumber=-8
  out16b : Outport
  wires:
  low/1 -> Data Type Conversion6/1
  Bitwise Operator2/1 -> out16b/1
  high/1 -> Data Type Conversion7/1
  Data Type Conversion7/1 -> Shift Arithmetic2/1
  Shift Arithmetic2/1 -> Bitwise Operator2/2
  Data Type Conversion6/1 -> Bitwise Operator2/1

== system CubeX/SPI3 get Data4/Turn the MSB and LSB into a signed 16-bit integer AccZ ==
  low : Inport
  high : Inport  Port=2
  Bitwise Operator2 : simulink/Logic and Bit Operations/Bitwise Operator  logicop=OR  UseBitMask=off  NumInputPorts=2  BitMask=bin2dec('11011001')  BitMaskRealWorld=Stored Integer
  Data Type Conversion6 : DataTypeConversion  OutDataTypeStr=uint16
  Data Type Conversion7 : DataTypeConversion  OutDataTypeStr=uint16
  Shift Arithmetic2 : ArithShift  BitShiftNumber=-8
  out16b : Outport
  wires:
  low/1 -> Data Type Conversion6/1
  Bitwise Operator2/1 -> out16b/1
  high/1 -> Data Type Conversion7/1
  Data Type Conversion7/1 -> Shift Arithmetic2/1
  Shift Arithmetic2/1 -> Bitwise Operator2/2
  Data Type Conversion6/1 -> Bitwise Operator2/1

== system CubeX/SPI3 get Data4/Turn the MSB and LSB into a signed 16-bit integer AccZ1 ==
  low : Inport
  high : Inport  Port=2
  Bitwise Operator2 : simulink/Logic and Bit Operations/Bitwise Operator  logicop=OR  UseBitMask=off  NumInputPorts=2  BitMask=bin2dec('11011001')  BitMaskRealWorld=Stored Integer
  Data Type Conversion6 : DataTypeConversion  OutDataTypeStr=uint16
  Data Type Conversion7 : DataTypeConversion  OutDataTypeStr=uint16
  Shift Arithmetic2 : ArithShift  BitShiftNumber=-8
  out16b : Outport
  wires:
  low/1 -> Data Type Conversion6/1
  Bitwise Operator2/1 -> out16b/1
  high/1 -> Data Type Conversion7/1
  Data Type Conversion7/1 -> Shift Arithmetic2/1
  Shift Arithmetic2/1 -> Bitwise Operator2/2
  Data Type Conversion6/1 -> Bitwise Operator2/1

== system CubeX/SPI3 get Data4/Turn the MSB and LSB into a signed 16-bit integer MagX ==
  low : Inport
  high : Inport  Port=2
  Bitwise Operator2 : simulink/Logic and Bit Operations/Bitwise Operator  logicop=OR  UseBitMask=off  NumInputPorts=2  BitMask=bin2dec('11011001')  BitMaskRealWorld=Stored Integer
  Data Type Conversion6 : DataTypeConversion  OutDataTypeStr=uint16
  Data Type Conversion7 : DataTypeConversion  OutDataTypeStr=uint16
  Shift Arithmetic2 : ArithShift  BitShiftNumber=-8
  out16b : Outport
  wires:
  low/1 -> Data Type Conversion6/1
  Bitwise Operator2/1 -> out16b/1
  high/1 -> Data Type Conversion7/1
  Data Type Conversion7/1 -> Shift Arithmetic2/1
  Shift Arithmetic2/1 -> Bitwise Operator2/2
  Data Type Conversion6/1 -> Bitwise Operator2/1

== system CubeX/SPI3 get Data4/Turn the MSB and LSB into a signed 16-bit integer MagY ==
  low : Inport
  high : Inport  Port=2
  Bitwise Operator2 : simulink/Logic and Bit Operations/Bitwise Operator  logicop=OR  UseBitMask=off  NumInputPorts=2  BitMask=bin2dec('11011001')  BitMaskRealWorld=Stored Integer
  Data Type Conversion6 : DataTypeConversion  OutDataTypeStr=uint16
  Data Type Conversion7 : DataTypeConversion  OutDataTypeStr=uint16
  Shift Arithmetic2 : ArithShift  BitShiftNumber=-8
  out16b : Outport
  wires:
  low/1 -> Data Type Conversion6/1
  Bitwise Operator2/1 -> out16b/1
  high/1 -> Data Type Conversion7/1
  Data Type Conversion7/1 -> Shift Arithmetic2/1
  Shift Arithmetic2/1 -> Bitwise Operator2/2
  Data Type Conversion6/1 -> Bitwise Operator2/1

== system CubeX/SPI3 get Data4/Turn the MSB and LSB into a signed 16-bit integer MagZ ==
  low : Inport
  high : Inport  Port=2
  Bitwise Operator2 : simulink/Logic and Bit Operations/Bitwise Operator  logicop=OR  UseBitMask=off  NumInputPorts=2  BitMask=bin2dec('11011001')  BitMaskRealWorld=Stored Integer
  Data Type Conversion6 : DataTypeConversion  OutDataTypeStr=uint16
  Data Type Conversion7 : DataTypeConversion  OutDataTypeStr=uint16
  Shift Arithmetic2 : ArithShift  BitShiftNumber=-8
  out16b : Outport
  wires:
  low/1 -> Data Type Conversion6/1
  Bitwise Operator2/1 -> out16b/1
  high/1 -> Data Type Conversion7/1
  Data Type Conversion7/1 -> Shift Arithmetic2/1
  Shift Arithmetic2/1 -> Bitwise Operator2/2
  Data Type Conversion6/1 -> Bitwise Operator2/1

== system CubeX/SPI3 get Data4/USE THIS ONE!!2 ==
  "Gyro_Zout_High " : Inport
  Gyro_Zout_Low : Inport  Port=2
  Bitwise Operator : simulink/Logic and Bit Operations/Bitwise Operator  logicop=OR  UseBitMask=off  NumInputPorts=2  BitMask=bin2dec('11011001')  BitMaskRealWorld=Stored Integer
  Data Type Conversion : DataTypeConversion  OutDataTypeStr=uint16
  Data Type Conversion1 : DataTypeConversion  OutDataTypeStr=uint16
  Shift Arithmetic : ArithShift  BitShiftNumber=-8
  Gyro_Zout : Outport
  wires:
  Gyro_Zout_Low/1 -> Data Type Conversion/1
  "Gyro_Zout_High "/1 -> Data Type Conversion1/1
  Data Type Conversion1/1 -> Shift Arithmetic/1
  Data Type Conversion/1 -> Bitwise Operator/2
  Shift Arithmetic/1 -> Bitwise Operator/1
  Bitwise Operator/1 -> Gyro_Zout/1

== system CubeX/SPI3 get Data4/USE THIS ONE!!3 ==
  "Gyro_Zout_High " : Inport
  Gyro_Zout_Low : Inport  Port=2
  Bitwise Operator : simulink/Logic and Bit Operations/Bitwise Operator  logicop=OR  UseBitMask=off  NumInputPorts=2  BitMask=bin2dec('11011001')  BitMaskRealWorld=Stored Integer
  Data Type Conversion : DataTypeConversion  OutDataTypeStr=uint16
  Data Type Conversion1 : DataTypeConversion  OutDataTypeStr=uint16
  Shift Arithmetic : ArithShift  BitShiftNumber=-8
  Gyro_Zout : Outport
  wires:
  Gyro_Zout_Low/1 -> Data Type Conversion/1
  "Gyro_Zout_High "/1 -> Data Type Conversion1/1
  Data Type Conversion1/1 -> Shift Arithmetic/1
  Data Type Conversion/1 -> Bitwise Operator/2
  Shift Arithmetic/1 -> Bitwise Operator/1
  Bitwise Operator/1 -> Gyro_Zout/1

== system CubeX/SPI3 get Data4/USE THIS ONE!!4 ==
  "Gyro_Zout_High " : Inport
  Gyro_Zout_Low : Inport  Port=2
  Bitwise Operator : simulink/Logic and Bit Operations/Bitwise Operator  logicop=OR  UseBitMask=off  NumInputPorts=2  BitMask=bin2dec('11011001')  BitMaskRealWorld=Stored Integer
  Data Type Conversion : DataTypeConversion  OutDataTypeStr=uint16
  Data Type Conversion1 : DataTypeConversion  OutDataTypeStr=uint16
  Shift Arithmetic : ArithShift  BitShiftNumber=-8
  Gyro_Zout : Outport
  wires:
  Gyro_Zout_Low/1 -> Data Type Conversion/1
  "Gyro_Zout_High "/1 -> Data Type Conversion1/1
  Data Type Conversion1/1 -> Shift Arithmetic/1
  Data Type Conversion/1 -> Bitwise Operator/2
  Shift Arithmetic/1 -> Bitwise Operator/1
  Bitwise Operator/1 -> Gyro_Zout/1

== matlab function CubeX/USB VCP Send/Sample counter ==
  data: sample output
function sample = SampleCounter
%#codegen

persistent sample_count;

if isempty(sample_count)
    sample_count = 0;
end

sample_count = sample_count + 1;

sample = sample_count;

== matlab function CubeX/Acc ==
  data: acc input size=[3 1]; acc_out output size=[3 1]; gyro input; gyro_out output
function [acc_out,gyro_out] = fcn(acc,gyro)

% Bodyframe = Sensorframe
%   Xb      =   Ys
%   Yb      =   -Zs
%   Zb      =   Xs


 R = [0.9603    0.0936   -0.2627
    0.0936    0.7794    0.6195
    0.2627   -0.6195    0.7397];

%R45x = [1.0000         0         0
%         0    0.7071    0.7071
%         0   -0.7071    0.7071];

%acc_out = zeros(3,1);
%gyro_out = zeros(3,1);

acc_out = acc;
gyro_out = gyro;

%acc_out(1) = acc(2);
%acc_out(2) = -acc(3);
%acc_out(3) = -acc(1);

%gyro_out(1) = gyro(2);
%gyro_out(2) = -gyro(3);
%gyro_out(3) = -gyro(1);

%acc_out = R *  acc_out;
%gyro_out = R *  gyro_out;

%acc_out = R45x * acc_out;
%gyro_out = R45x * gyro_out;

== matlab function CubeX/MATLAB Function ==
  data: acc input; q output; gyro input
function q = Magdwick(acc,gyro)

    persistent AHRS;
    
    if isempty(AHRS)      
       AHRS = MadgwickAHRS('SamplePeriod', 1/500, 'Beta', 0.1); 
    end
    AHRS.UpdateIMU(gyro, acc);
    q = AHRS.Quaternion;

== matlab function CubeX/SPI3 get Data4/Take away Sensor fail reading ==
  data: y output; new input; old input
function y = fcn(new, old)
%#codegen
if(new > -257 && new < -200)
   y = old;
else
    y = new;
end

== matlab function CubeX/SPI3 get Data4/Take away Sensor fail reading if two bad in raw ==
  data: y output; new input; old input
function y = fcn(new, old)
%#codegen
if(new > -257 && new < -200)
   y = old;
else
    y = new;
end

== matlab function CubeX/SPI3 get Data4/Take away Sensor fail reading if two bad in raw1 ==
  data: y output; new input; old input
function y = fcn(new, old)
%#codegen
if(new > -257 && new < -200)
   y = old;
else
    y = new;
end

== matlab function CubeX/SPI3 get Data4/Take away Sensor fail reading1 ==
  data: y output; new input; old input
function y = fcn(new, old)
%#codegen
if(new > -257 && new < -200)
   y = old;
else
    y = new;
end
